simulink model "sampleModel221"  (R2021b)
settings: Solver=VariableStepAuto  StartTime=0.0  StopTime=10.0  RelTol=1e-3
undefined symbols (not defined in the file or in its folder): DiscIntNeverNeededParam
libraries: simulink x6
settings Model: Creator=user  LastModifiedBy=user

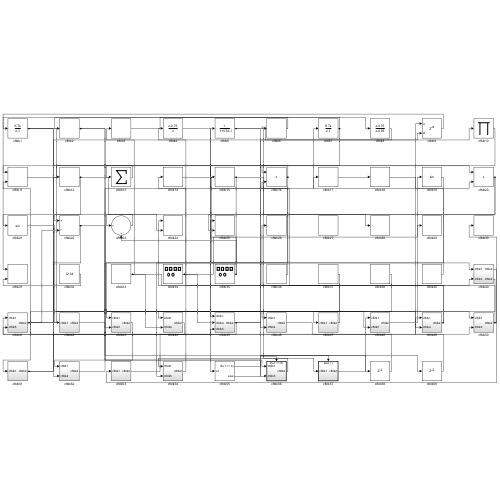
[thumbnail: Simulink's stored preview of the top-level diagram]
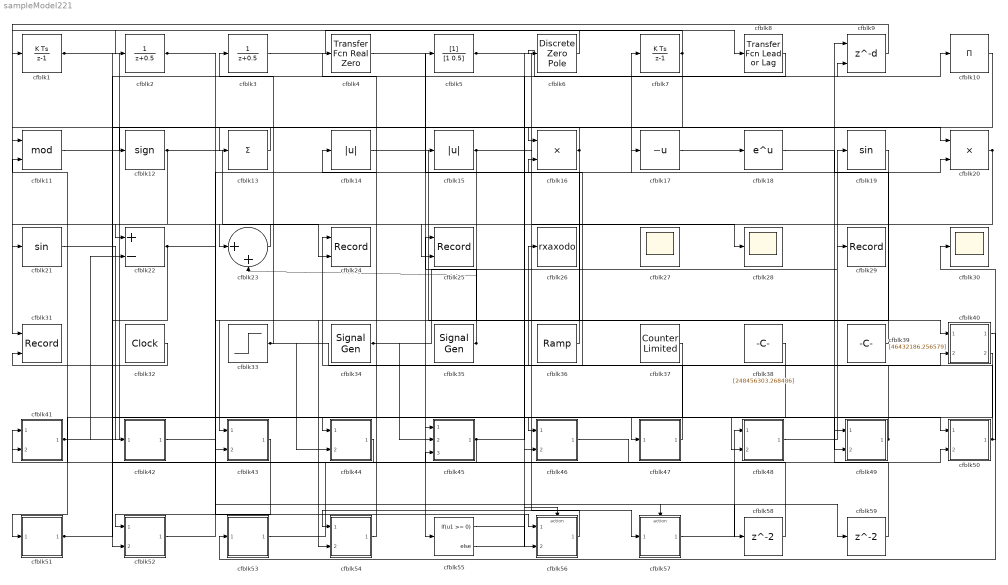
== system sampleModel221 ==
  cfblk1 : DiscreteIntegrator  ICPrevOutput=DiscIntNeverNeededParam  ICPrevScaledInput=DiscIntNeverNeededParam
  cfblk10 : Product  Inputs=*
  cfblk11 : Math  Operator=mod  SaturateOnIntegerOverflow=on
  cfblk12 : Signum
  cfblk13 : Sum  Inputs=+
  cfblk14 : Abs
  cfblk15 : Abs
  cfblk16 : Product
  cfblk17 : UnaryMinus
  cfblk18 : Math  SaturateOnIntegerOverflow=on
  cfblk19 : Trigonometry
  cfblk2 : DiscreteTransferFcn  SampleTime=1
  cfblk20 : Product  Inputs=**
  cfblk21 : Trigonometry
  cfblk22 : Sum  Inputs=+-
  cfblk23 : Sum  Inputs=|++
  cfblk24 : Record  FileSettingsInternal="{\"entries\":[{\"content\":{\"excelSettings\":{\"content\":{},\"type\":\"Streamout.ExcelSettings\"}},\"type\":\"Streamout.FileSettingStorage\",\"uuid\":\"17b5df4e-5c45-4ce3-adcc-850265834236\"}],\"packageUris\":[\"http://schema.mathworks.com/mf0/streamout_blocks/R2020a\"],\"version\":\"1.0\"}"  Layout=[1 1]  SignalsInternal="{\"entries\":[{\"content\":{\"signals\":[{\"content\":{\"blockPath\":[\"sampleModel221/cfblk24\"],\"channel\":[],\"dimensions\":[1],\"domain\":\"sampleModel221/cfblk24\",\"lineColor\":\"#a2142f\",\"plots\":[1],\"port\":1,\"sid\":[\"\"],\"signalID\":8606,\"signalName\":\"cfblk47\"},\"type\":\"RecordBlkView.Signal\",\"uuid\":\"ef50f66b-ef1e-4f28-aa92-86302d7e572f\"},{\"content\":{\"blockPath\":[\"sampleModel221/cfblk24\"],\"channel\":[],\"dimensions\":[1],\"domain\":\"sampleModel221/cfblk24\",\"lineColor\":\"#139fff\",\"plots\":[1],\"port\":2,\"sid\":[\"\"],\"signalID\":8610,\"signalName\":\"cfblk12\"},\"type\":\"RecordBlkView.Signal\",\"uuid\":\"b42bac8e-8f74-4232-b8c7-8db795f1838c\"}]},\"type\":\"RecordBlkView.InputSignals\",\"uuid\":\"97930701-0daf-4181-9298-0a435e11c254\"}],\"packageUris\":[\"http://schema.mathworks.com/mf0/streamout_blocks/R2020a\"],\"version\":\"1.0\"}"  VisualizationBindings="{\"xyplotplugin\":{\"info\":[{\"series\":[{\"bindingParametersList\":[{\"parameter\":\"X-Axis\",\"signalID\":8606,\"signalName\":\"cfblk47\"},{\"parameter\":\"Y-Axis\",\"signalID\":8610,\"signalName\":\"cfblk12\"}],\"seriesID\":43849}],\"subplotID\":1}]}}"  CompatibilityTag=XY
  cfblk25 : Record  FileSettingsInternal="{\"entries\":[{\"content\":{\"excelSettings\":{\"content\":{},\"type\":\"Streamout.ExcelSettings\"}},\"type\":\"Streamout.FileSettingStorage\",\"uuid\":\"71e33b4c-764c-4138-a6ed-e1cbbb26cc10\"}],\"packageUris\":[\"http://schema.mathworks.com/mf0/streamout_blocks/R2020a\"],\"version\":\"1.0\"}"  Layout=[1 1]  SignalsInternal="{\"entries\":[{\"content\":{\"signals\":[{\"content\":{\"blockPath\":[\"sampleModel221/cfblk25\"],\"channel\":[],\"dimensions\":[1],\"domain\":\"sampleModel221/cfblk25\",\"lineColor\":\"#a2142f\",\"plots\":[1],\"port\":1,\"sid\":[\"\"],\"signalID\":8614,\"signalName\":\"cfblk35\"},\"type\":\"RecordBlkView.Signal\",\"uuid\":\"355ad24c-c70a-4d4e-91a4-ae64254e8cec\"},{\"content\":{\"blockPath\":[\"sampleModel221/cfblk25\"],\"channel\":[],\"dimensions\":[1],\"domain\":\"sampleModel221/cfblk25\",\"lineColor\":\"#139fff\",\"plots\":[1],\"port\":2,\"sid\":[\"\"],\"signalID\":8618,\"signalName\":\"cfblk20\"},\"type\":\"RecordBlkView.Signal\",\"uuid\":\"3a16174d-c924-402c-ad84-5d5c20e9b461\"}]},\"type\":\"RecordBlkView.InputSignals\",\"uuid\":\"9fc8c057-8523-4a67-8aef-ab72b17a4c0c\"}],\"packageUris\":[\"http://schema.mathworks.com/mf0/streamout_blocks/R2020a\"],\"version\":\"1.0\"}"  VisualizationBindings="{\"xyplotplugin\":{\"info\":[{\"series\":[{\"bindingParametersList\":[{\"parameter\":\"X-Axis\",\"signalID\":8614,\"signalName\":\"cfblk35\"},{\"parameter\":\"Y-Axis\",\"signalID\":8618,\"signalName\":\"cfblk20\"}],\"seriesID\":4177}],\"subplotID\":1}]}}"  CompatibilityTag=XY
  cfblk26 : ToWorkspace  VariableName=rxaxodo  SaveFormat=Timeseries  SampleTime=-1
  cfblk27 : Scope
      settings: Floating=on
  cfblk28 : Scope
  cfblk29 : Record  FileSettingsInternal="{\"entries\":[{\"content\":{\"excelSettings\":{\"content\":{},\"type\":\"Streamout.ExcelSettings\"}},\"type\":\"Streamout.FileSettingStorage\",\"uuid\":\"4d7a7f12-0234-42ac-a42e-fb5ca3b5d160\"}],\"packageUris\":[\"http://schema.mathworks.com/mf0/streamout_blocks/R2020a\"],\"version\":\"1.0\"}"  SignalsInternal="{\"entries\":[{\"content\":{\"signals\":[{\"content\":{\"blockPath\":[\"sampleModel221/cfblk29\"],\"channel\":[],\"dimensions\":[1],\"domain\":\"sampleModel221/cfblk29\",\"lineColor\":\"#a2142f\",\"plots\":[1],\"port\":1,\"sid\":[\"\"],\"signalID\":8622,\"signalName\":\"cfblk34\"},\"type\":\"RecordBlkView.Signal\",\"uuid\":\"5069e872-126a-497e-beef-7b01c2a22045\"}]},\"type\":\"RecordBlkView.InputSignals\",\"uuid\":\"ab89346d-cc94-4e93-86bf-061923d18382\"}],\"packageUris\":[\"http://schema.mathworks.com/mf0/streamout_blocks/R2020a\"],\"version\":\"1.0\"}"  VisualizationBindings="{\"sparklinesplugin\":{\"info\":[{\"bindingParametersList\":[],\"subplotID\":1}]}}"
  cfblk3 : DiscreteTransferFcn  SampleTime=1
  cfblk30 : Scope
  cfblk31 : Record  FileSettingsInternal="{\"entries\":[{\"content\":{\"excelSettings\":{\"content\":{},\"type\":\"Streamout.ExcelSettings\"}},\"type\":\"Streamout.FileSettingStorage\",\"uuid\":\"7a72385a-f96f-4a12-929e-36e116d166a0\"}],\"packageUris\":[\"http://schema.mathworks.com/mf0/streamout_blocks/R2020a\"],\"version\":\"1.0\"}"  Layout=[1 1]  SignalsInternal="{\"entries\":[{\"content\":{\"signals\":[{\"content\":{\"blockPath\":[\"sampleModel221/cfblk31\"],\"channel\":[],\"dimensions\":[1],\"domain\":\"sampleModel221/cfblk31\",\"lineColor\":\"#a2142f\",\"plots\":[1],\"port\":1,\"sid\":[\"\"],\"signalID\":8626,\"signalName\":\"cfblk9\"},\"type\":\"RecordBlkView.Signal\",\"uuid\":\"a96c8959-c816-4740-a9c3-f827df62f38c\"},{\"content\":{\"blockPath\":[\"sampleModel221/cfblk31\"],\"channel\":[],\"dimensions\":[1],\"domain\":\"sampleModel221/cfblk31\",\"lineColor\":\"#139fff\",\"plots\":[1],\"port\":2,\"sid\":[\"\"],\"signalID\":8630,\"signalName\":\"cfblk32\"},\"type\":\"RecordBlkView.Signal\",\"uuid\":\"e11e56f3-1ada-4e8a-ad92-bbcd29de4942\"}]},\"type\":\"RecordBlkView.InputSignals\",\"uuid\":\"185051c9-ffca-467c-94e2-2aa00d9344ec\"}],\"packageUris\":[\"http://schema.mathworks.com/mf0/streamout_blocks/R2020a\"],\"version\":\"1.0\"}"  VisualizationBindings="{\"xyplotplugin\":{\"info\":[{\"series\":[{\"bindingParametersList\":[{\"parameter\":\"X-Axis\",\"signalID\":8626,\"signalName\":\"cfblk9\"},{\"parameter\":\"Y-Axis\",\"signalID\":8630,\"signalName\":\"cfblk32\"}],\"seriesID\":59212}],\"subplotID\":1}]}}"  CompatibilityTag=XY
  cfblk32 : DigitalClock
  cfblk33 : Step  Time=[5.000000]  Before=[-908870727.442737]  After=[586403943.823782]  SampleTime=0
  cfblk34 : SignalGenerator  Amplitude=[-209875020.457807]  Units=rad/sec
  cfblk35 : SignalGenerator  Amplitude=[816065188.618249]
  cfblk36 : simulink/Sources/Ramp  slope=[-1461.633410]  start=[2.450126]  InitialOutput=[-589045.849010]
  cfblk37 : simulink/Sources/Counter Limited  uplimit=[311.000000]  tsamp=-1
  cfblk38 : Constant  Value=[248456303.268486]  SampleTime=1
  cfblk39 : Constant  Value=[46432186.256579]  SampleTime=1
  cfblk4 : simulink/Discrete/Transfer Fcn Real Zero  ZeroZ=0.75  ICPrevInput=0.0  DoSatur=off
      settings: SourceProductBaseCode=SL
  cfblk40 : Subsystem
  cfblk41 : Subsystem
  cfblk42 : Subsystem
  cfblk43 : Subsystem
  cfblk44 : Subsystem
  cfblk45 : Subsystem
  cfblk46 : Subsystem
  cfblk47 : Subsystem
  cfblk48 : Subsystem
  cfblk49 : Subsystem
  cfblk5 : DiscreteFilter  SampleTime=1
  cfblk50 : Subsystem
  cfblk51 : Subsystem
  cfblk52 : Subsystem
  cfblk53 : Subsystem
  cfblk54 : Subsystem
  cfblk55 : If  IfExpression=u1 >= 0  SampleTime=1
  cfblk56 : Subsystem  TreatAsAtomicUnit=on
  cfblk57 : Subsystem  TreatAsAtomicUnit=on
  cfblk58 : Delay  SampleTime=1
  cfblk59 : Delay  SampleTime=1
  cfblk6 : DiscreteZeroPole  Poles=[0 0.5]  Gain=1
  cfblk7 : DiscreteIntegrator  ICPrevOutput=DiscIntNeverNeededParam  ICPrevScaledInput=DiscIntNeverNeededParam
  cfblk8 : simulink/Discrete/Transfer Fcn Lead or Lag  PoleZ=0.95  ZeroZ=0.75  ICPrevOutput=0.0  ICPrevInput=0.0  DoSatur=off
      settings: SourceProductBaseCode=SL
  cfblk9 : Delay  DelayLengthSource=Input port  SampleTime=1
      settings: InputPortMap=u0,p1
  wires:
  cfblk3/1 -> cfblk8/1
  cfblk41/1(cfblk2) -> cfblk50/1(cfblk1), cfblk22/2, cfblk10/1
  cfblk5/1 -> cfblk57/1(cfblk1), cfblk48/2(cfblk5)
  cfblk9/1 -> cfblk31/1
  cfblk13/1 -> cfblk11/1
  cfblk47/1(cfblk2) -> cfblk24/1
  cfblk48/1(cfblk2) -> cfblk19/1
  cfblk44/1(cfblk2) -> cfblk41/1(cfblk1)
  cfblk45/1(cfblk2) -> cfblk41/2(cfblk5), cfblk9/2, cfblk59/1
  cfblk12/1 -> cfblk24/2, cfblk22/1
  cfblk20/1 -> cfblk23/1, cfblk25/2
  cfblk40/1(cfblk2) -> cfblk53/1(cfblk1)
  cfblk38/1 -> cfblk51/1(cfblk1)
  cfblk8/1 -> cfblk6/1
  cfblk1/1 -> cfblk46/1(cfblk1), cfblk15/1, cfblk46/2(cfblk4)
  cfblk15/1 -> cfblk43/1(cfblk1), cfblk28/1
  cfblk7/1 -> cfblk55/1, cfblk2/1
  cfblk23/1 -> cfblk21/1
  cfblk39/1 -> cfblk7/1
  cfblk40/2(cfblk4) -> cfblk47/1(cfblk1)
  cfblk37/1 -> cfblk44/1(cfblk1)
  cfblk53/1(cfblk2) -> cfblk9/1
  cfblk19/1 -> cfblk43/2(cfblk3)
  cfblk17/1 -> cfblk18/1
  cfblk14/1 -> cfblk40/1(cfblk1)
  cfblk22/1 -> cfblk56/1(cfblk1), cfblk52/2(cfblk4)
  cfblk16/1 -> cfblk13/1, cfblk54/2(cfblk5)
  cfblk52/1(cfblk2) -> cfblk17/1
  cfblk11/1 -> cfblk20/1
  cfblk50/1(cfblk2) -> cfblk30/1, cfblk16/2
  cfblk10/1 -> cfblk16/1
  cfblk33/1 -> cfblk3/1, cfblk40/2(cfblk3), cfblk44/2(cfblk4)
  cfblk43/1(cfblk2) -> cfblk52/1(cfblk1)
  cfblk2/1 -> cfblk49/2(cfblk4), cfblk56/2(cfblk3)
  cfblk49/1(cfblk2) -> cfblk26/1, cfblk4/1
  cfblk54/1(cfblk2) -> cfblk14/1
  cfblk18/1 -> cfblk20/2
  cfblk46/1(cfblk2) -> cfblk50/2(cfblk3)
  cfblk4/1 -> cfblk45/1(cfblk1)
  cfblk21/1 -> cfblk42/1(cfblk1)
  cfblk34/1 -> cfblk29/1, cfblk45/2(cfblk4)
  cfblk32/1 -> cfblk31/2
  cfblk6/1 -> cfblk1/1
  cfblk35/1 -> cfblk23/2, cfblk25/1
  cfblk56/1(cfblk2) -> cfblk54/1(cfblk1)
  cfblk57/1(cfblk2) -> cfblk48/1(cfblk1)
  cfblk36/1 -> cfblk5/1
  cfblk51/1(cfblk2) -> cfblk12/1, cfblk45/3(cfblk5)
  cfblk55/1 -> cfblk56/Action
  cfblk55/2 -> cfblk57/Action
  cfblk42/1(cfblk2) -> cfblk58/1
  cfblk58/1 -> cfblk11/2
  cfblk59/1 -> cfblk49/1(cfblk1)

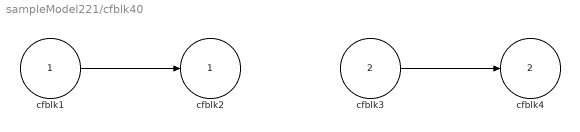
== system sampleModel221/cfblk40 ==
  cfblk1 : Inport
  cfblk3 : Inport  Port=2
  cfblk2 : Outport
  cfblk4 : Outport  Port=2
  wires:
  cfblk1/1 -> cfblk2/1
  cfblk3/1 -> cfblk4/1

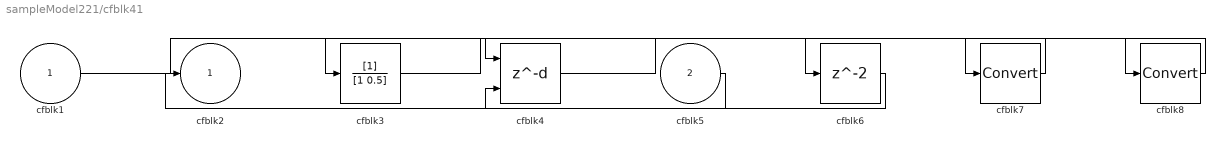
== system sampleModel221/cfblk41 ==
  cfblk1 : Inport
  cfblk5 : Inport  Port=2
  cfblk3 : DiscreteFilter  SampleTime=1
  cfblk4 : Delay  DelayLengthSource=Input port  SampleTime=1
      settings: InputPortMap=u0,p1
  cfblk6 : Delay  SampleTime=1
  cfblk7 : DataTypeConversion
  cfblk8 : DataTypeConversion
  cfblk2 : Outport
  wires:
  cfblk1/1 -> cfblk4/1
  cfblk5/1 -> cfblk2/1
  cfblk6/1 -> cfblk4/2
  cfblk3/1 -> cfblk7/1
  cfblk7/1 -> cfblk6/1
  cfblk4/1 -> cfblk8/1
  cfblk8/1 -> cfblk3/1

== system sampleModel221/cfblk42 ==
  cfblk1 : Inport
  cfblk3 : Constant  Value=[385128852.901008]  SampleTime=1
  cfblk2 : Outport
  wires:
  cfblk3/1 -> cfblk2/1

== system sampleModel221/cfblk43 ==
  cfblk1 : Inport
  cfblk3 : Inport  Port=2
  cfblk2 : Outport
  wires:
  cfblk3/1 -> cfblk2/1

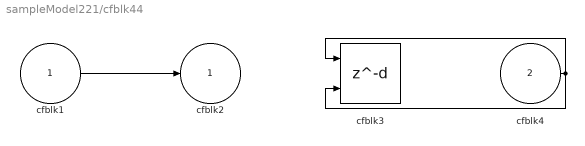
== system sampleModel221/cfblk44 ==
  cfblk1 : Inport
  cfblk4 : Inport  Port=2
  cfblk3 : Delay  DelayLengthSource=Input port  SampleTime=1
      settings: InputPortMap=u0,p1
  cfblk2 : Outport
  wires:
  cfblk1/1 -> cfblk2/1
  cfblk4/1 -> cfblk3/1, cfblk3/2

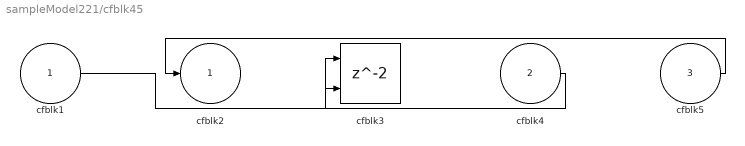
== system sampleModel221/cfblk45 ==
  cfblk1 : Inport
  cfblk4 : Inport  Port=2
  cfblk5 : Inport  Port=3
  cfblk3 : Delay  ShowEnablePort=on  SampleTime=1
      settings: InputPortMap=u0,e6
  cfblk2 : Outport
  wires:
  cfblk5/1 -> cfblk2/1
  cfblk1/1 -> cfblk3/1
  cfblk4/1 -> cfblk3/2

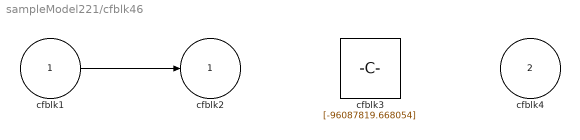
== system sampleModel221/cfblk46 ==
  cfblk1 : Inport
  cfblk4 : Inport  Port=2
  cfblk3 : Constant  Value=[-96087819.668054]  SampleTime=1
  cfblk2 : Outport
  wires:
  cfblk1/1 -> cfblk2/1

== system sampleModel221/cfblk47 ==
  cfblk1 : Inport
  cfblk3 : Reshape
  cfblk2 : Outport
  wires:
  cfblk1/1 -> cfblk3/1
  cfblk3/1 -> cfblk2/1

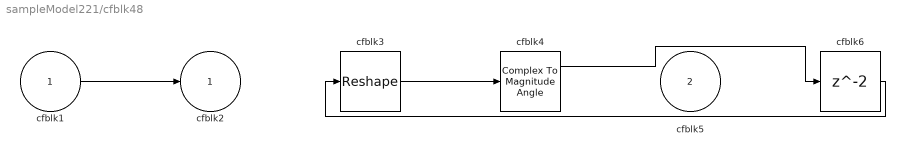
== system sampleModel221/cfblk48 ==
  cfblk1 : Inport
  cfblk5 : Inport  Port=2
  cfblk3 : Reshape
  cfblk4 : ComplexToMagnitudeAngle
  cfblk6 : Delay  SampleTime=1
  cfblk2 : Outport
  wires:
  cfblk3/1 -> cfblk4/1
  cfblk1/1 -> cfblk2/1
  cfblk4/1 -> cfblk6/1
  cfblk6/1 -> cfblk3/1

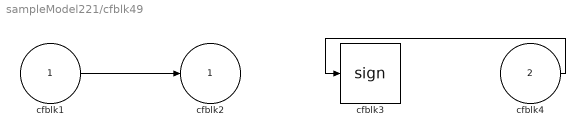
== system sampleModel221/cfblk49 ==
  cfblk1 : Inport
  cfblk4 : Inport  Port=2
  cfblk3 : Signum
  cfblk2 : Outport
  wires:
  cfblk4/1 -> cfblk3/1
  cfblk1/1 -> cfblk2/1

== system sampleModel221/cfblk50 ==
  cfblk1 : Inport
  cfblk3 : Inport  Port=2
  cfblk2 : Outport
  wires:
  cfblk1/1 -> cfblk2/1

== system sampleModel221/cfblk51 ==
  cfblk1 : Inport
  cfblk3 : MinMax  Function=max
  cfblk2 : Outport
  wires:
  cfblk1/1 -> cfblk2/1, cfblk3/1

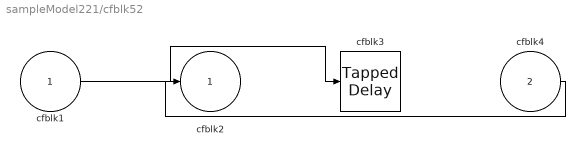
== system sampleModel221/cfblk52 ==
  cfblk1 : Inport
  cfblk4 : Inport  Port=2
  cfblk3 : simulink/Discrete/Tapped Delay  vinit=0.0  samptime=-1  NumDelays=1  DelayOrder=Oldest  includeCurrent=off
  cfblk2 : Outport
  wires:
  cfblk1/1 -> cfblk3/1
  cfblk4/1 -> cfblk2/1

== system sampleModel221/cfblk53 ==
  cfblk1 : Inport
  cfblk3 : simulink/Discrete/Difference  ICPrevInput=0.0  OutMin=[]  OutMax=[]  OutDataTypeStr=Inherit: Inherit via back propagation  OutDataType=fixdt(1, 16)  OutScaling=2^-10  DoSatur=off
  cfblk2 : Outport
  wires:
  cfblk1/1 -> cfblk3/1
  cfblk3/1 -> cfblk2/1

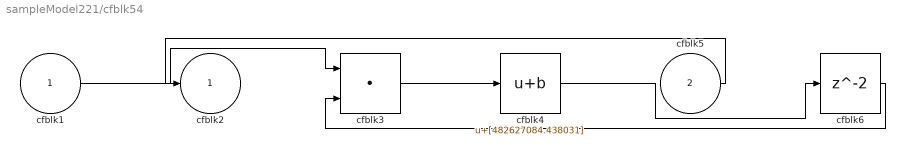
== system sampleModel221/cfblk54 ==
  cfblk1 : Inport
  cfblk5 : Inport  Port=2
  cfblk3 : DotProduct  InputSameDT=on  OutDataTypeStr=Inherit: Inherit via internal rule
  cfblk4 : Bias  Bias=[482627084.438031]
  cfblk6 : Delay  SampleTime=1
  cfblk2 : Outport
  wires:
  cfblk1/1 -> cfblk3/1
  cfblk3/1 -> cfblk4/1
  cfblk5/1 -> cfblk2/1
  cfblk4/1 -> cfblk6/1
  cfblk6/1 -> cfblk3/2

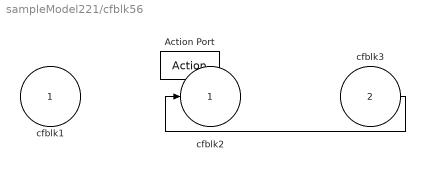
== system sampleModel221/cfblk56 ==
  cfblk1 : Inport
  cfblk3 : Inport  Port=2
  Action Port : ActionPort  ActionPortLabel=if(u1 >= 0)
  cfblk2 : Outport
  wires:
  cfblk3/1 -> cfblk2/1

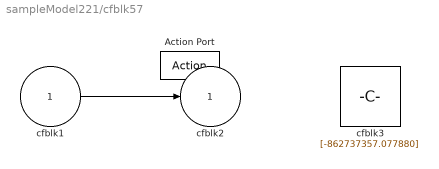
== system sampleModel221/cfblk57 ==
  cfblk1 : Inport
  Action Port : ActionPort  ActionPortLabel=else
  cfblk3 : Constant  Value=[-862737357.077880]  SampleTime=1
  cfblk2 : Outport
  wires:
  cfblk1/1 -> cfblk2/1
